simulink model "reactionWheel"  (R2019a)
settings: Solver=VariableStepAuto  StartTime=0.0  StopTime=20  RelTol=1e-3
model workspace (MAT data in the model file):
  Omega_max = 0.5
undefined symbols (not defined in the file or in its folder): sat, sigbuilder_block
libraries: simulink x3
settings Model: Creator=brice  LastModifiedBy=robin

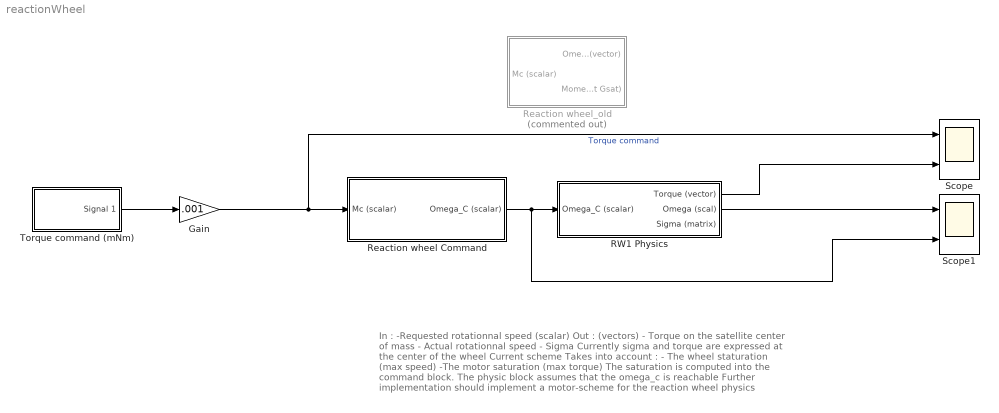
== system reactionWheel ==
  note: In :
      | -Requested rotationnal speed (scalar)
      | Out : (vectors)
      | - Torque on the satellite center of mass
      | - Actual rotationnal speed
      | - Sigma
      | Currently sigma and torque are expressed at the center of the wheel
      |
      | Current scheme
      | Takes into account :
      | - The wheel staturation (max speed)
      | -The motor saturation (max torque)
      |
      | The saturation is computed into the command block. The physic block assumes that the omega_c is reachable
      | Further implementation should implement a motor-scheme for the reaction wheel physics
  Gain : Gain  Gain=.001
  RW1 Physics : Subsystem
  Reaction wheel Command : Subsystem
  Reaction wheel_old : Subsystem  Commented=on
  Scope : Scope  NumInputPorts=2
  Scope1 : Scope  NumInputPorts=2
  Torque command (mNm) : Subsystem  Tag=STV Subsys  LoadFcn=sigbuilder_block('load');  StartFcn=sigbuilder_block('start');  StopFcn=sigbuilder_block('stop');  ClipboardFcn=sigbuilder_block('clipboard');  mask(Sigbuilder block){tuvar=[0:10]}
      mask help: Simulink:masks:SigbuilderBlock_MD
      mask init:
      | if ~strcmp(get_param(bdroot(gcbh),'SimulationStatus'),'stopped') tuvar = sigbuilder_block('maskInit'); end
      settings: CopyFcn=sigbuilder_block('copy');  DeleteFcn=sigbuilder_block('delete');  ModelCloseFcn=sigbuilder_block('modelClose');  PreSaveFcn=sigbuilder_block('preSave');  PauseFcn=sigbuilder_block('pause');  ContinueFcn=sigbuilder_block('continue');  NameChangeFcn=sigbuilder_block('namechange');  OpenFcn=sigbuilder_block('open',[437.6 199.2 604.15 400 ]);  CloseFcn=sigbuilder_block('close');
      mask Display: plot(0, 0, 100, 100,[2, 2, 32, 32, 2], [68, 8, 8, 68, 68],[32, 2], [38, 38], [32, 19, 2],[53, 60, 44], [32, 17, 17, 2],[16, 16, 31, 31]);txt = getActiveGroup(gcbh);text(2, 100, txt,'verticalAlignment', 'top');
  wires:
  Reaction wheel Command/1(Omega_C (scalar)) -> RW1 Physics/1(Omega_C (scalar)), Scope1/2
  Torque command (mNm)/1(Signal 1) -> Gain/1
  RW1 Physics/1(Torque (vector)) -> Scope/2
  Gain/1 -> Scope/1, Reaction wheel Command/1(Mc (scalar))  "Torque command"
  RW1 Physics/2(Omega (scal)) -> Scope1/1

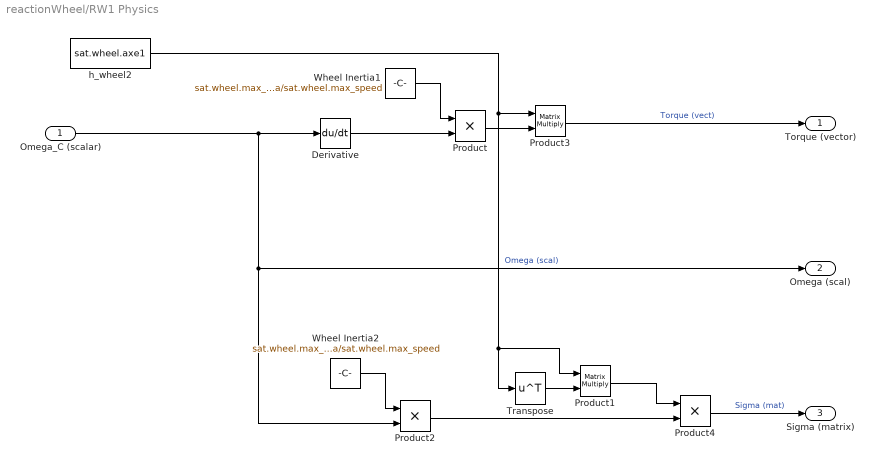
== system reactionWheel/RW1 Physics ==
  Omega_C (scalar) : Inport
  Derivative : Derivative
  Product : Product
  Product1 : Product  Multiplication=Matrix(*)
  Product2 : Product
  Product3 : Product  Multiplication=Matrix(*)
  Product4 : Product
  Transpose : Math  Operator=transpose  SaturateOnIntegerOverflow=on
  Wheel Inertia1 : Constant  Value=sat.wheel.max_sigma/sat.wheel.max_speed
  Wheel Inertia2 : Constant  Value=sat.wheel.max_sigma/sat.wheel.max_speed
  h_wheel2 : Constant  Value=sat.wheel.axe1
  Torque (vector) : Outport  VectorParamsAs1DForOutWhenUnconnected=on
  Omega (scal) : Outport  Port=2  VectorParamsAs1DForOutWhenUnconnected=on
  Sigma (matrix) : Outport  Port=3  VectorParamsAs1DForOutWhenUnconnected=on
  wires:
  Product3/1 -> Torque (vector)/1  "Torque (vect)"
  Wheel Inertia1/1 -> Product/1
  Omega_C (scalar)/1 -> Product2/2, Omega (scal)/1, Derivative/1  "Omega (scal)"
  Derivative/1 -> Product/2
  Product/1 -> Product3/2
  Wheel Inertia2/1 -> Product2/1
  Product4/1 -> Sigma (matrix)/1  "Sigma (mat)"
  Product2/1 -> Product4/2
  h_wheel2/1 -> Transpose/1, Product1/1, Product3/1
  Product1/1 -> Product4/1
  Transpose/1 -> Product1/2

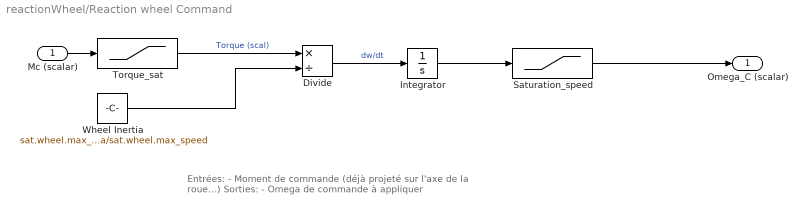
== system reactionWheel/Reaction wheel Command ==
  note: Entrées:
      | - Moment de commande (déjà projeté sur l'axe de la roue...)
      | Sorties:
      | - Omega de commande à appliquer
  Mc (scalar) : Inport
  Divide : Product  Inputs=*/
  Integrator : Integrator
  Saturation_speed : Saturate  UpperLimit=sat.wheel.max_speed  LowerLimit=- sat.wheel.max_speed
  Torque_sat : Saturate  UpperLimit=sat.wheel.max_torque  LowerLimit=- sat.wheel.max_torque
  Wheel Inertia : Constant  Value=sat.wheel.max_sigma/sat.wheel.max_speed
  Omega_C (scalar) : Outport  VectorParamsAs1DForOutWhenUnconnected=on
  wires:
  Mc (scalar)/1 -> Torque_sat/1
  Wheel Inertia/1 -> Divide/2
  Divide/1 -> Integrator/1  "dw/dt"
  Integrator/1 -> Saturation_speed/1
  Torque_sat/1 -> Divide/1  "Torque (scal)"
  Saturation_speed/1 -> Omega_C (scalar)/1

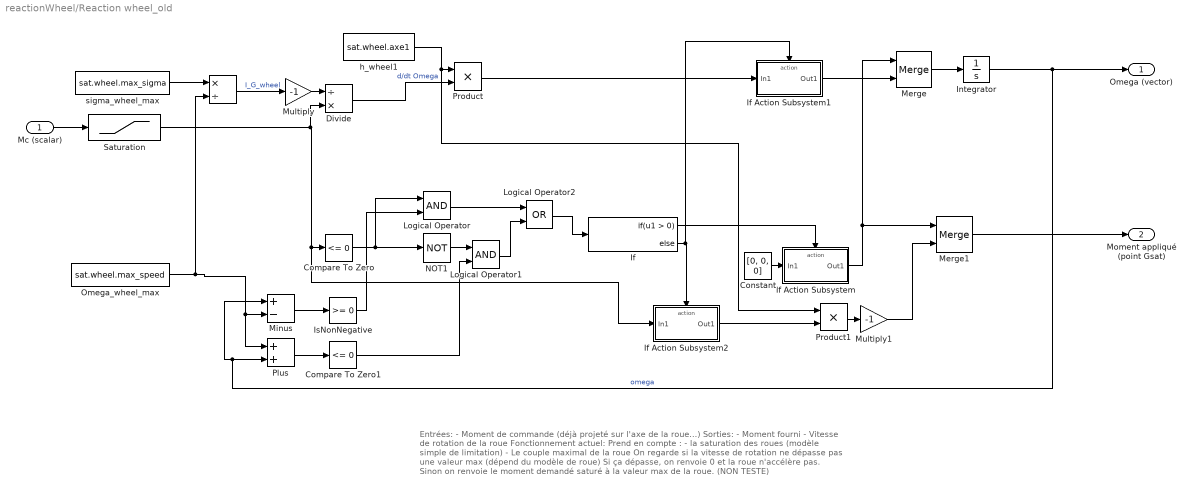
== system reactionWheel/Reaction wheel_old ==
  note: Entrées:
      | - Moment de commande (déjà projeté sur l'axe de la roue...)
      | Sorties:
      | - Moment fourni
      | - Vitesse de rotation de la roue
      |
      | Fonctionnement actuel:
      | Prend en compte :
      | - la saturation des roues (modèle simple de limitation)
      | - Le couple maximal de la roue
      |
      |
      | On regarde si la vitesse de rotation ne dépasse pas une valeur max (dépend du modèle de roue)
      | Si ça dépasse, on renvoie 0 et la roue n'accélère pas.
      | Sinon on renvoie le moment demandé saturé à la valeur max de la roue.
      |
      | (NON TESTE)
  Mc (scalar) : Inport
  " " : Product  Inputs=*/
  Compare To Zero : simulink/Logic and Bit Operations/Compare To Zero  relop=<=  OutDataTypeStr=boolean
  Compare To Zero1 : simulink/Logic and Bit Operations/Compare To Zero  relop=<=  OutDataTypeStr=boolean
  Constant : Constant  Value=[0, 0, 0]
  Divide : Product  Inputs=/*
  If : If
  If Action Subsystem : Subsystem  TreatAsAtomicUnit=on
  If Action Subsystem1 : Subsystem  TreatAsAtomicUnit=on
  If Action Subsystem2 : Subsystem  TreatAsAtomicUnit=on
  Integrator : Integrator
  IsNonNegative : simulink/Logic and Bit Operations/Compare To Zero  relop=>=  OutDataTypeStr=boolean
  Logical Operator : Logic  AllPortsSameDT=off  OutDataTypeStr=boolean
  Logical Operator1 : Logic  AllPortsSameDT=off  OutDataTypeStr=boolean
  Logical Operator2 : Logic  Operator=OR  AllPortsSameDT=off  OutDataTypeStr=boolean
  Merge : Merge
  Merge1 : Merge
  Minus : Sum  Inputs=+-
  Multiply : Gain  Gain=-1
  Multiply1 : Gain  Gain=-1
  NOT1 : Logic  Operator=NOT  IconShape=distinctive  AllPortsSameDT=off  OutDataTypeStr=boolean
  Omega_wheel_max : Constant  Value=sat.wheel.max_speed
  Plus : Sum
  Product : Product
  Product1 : Product
  Saturation : Saturate  UpperLimit=sat.wheel.max_torque  LowerLimit=- sat.wheel.max_torque
  h_wheel1 : Constant  Value=sat.wheel.axe1
  sigma_wheel_max : Constant  Value=sat.wheel.max_sigma
  Omega (vector) : Outport  VectorParamsAs1DForOutWhenUnconnected=on
  Moment appliqué (point Gsat) : Outport  Port=2  VectorParamsAs1DForOutWhenUnconnected=on
  wires:
  Integrator/1 -> Omega (vector)/1, Minus/1, Plus/2  "omega"
  If/2 -> If Action Subsystem2/Action, If Action Subsystem1/Action
  Saturation/1 -> If Action Subsystem2/1(In1), Compare To Zero/1, Divide/2
  IsNonNegative/1 -> Logical Operator/2
  Constant/1 -> If Action Subsystem/1(In1)
  Compare To Zero/1 -> Logical Operator/1, NOT1/1
  Divide/1 -> Product/2  "d/dt Omega"
  NOT1/1 -> Logical Operator1/1
  Omega_wheel_max/1 -> Plus/1, Minus/2, " "/2
  Logical Operator2/1 -> If/1
  If/1 -> If Action Subsystem/Action
  Product/1 -> If Action Subsystem1/1(In1)
  If Action Subsystem/1(Out1) -> Merge1/1, Merge/1
  Minus/1 -> IsNonNegative/1
  Compare To Zero1/1 -> Logical Operator1/2
  Plus/1 -> Compare To Zero1/1
  If Action Subsystem1/1(Out1) -> Merge/2
  Merge1/1 -> Moment appliqué (point Gsat)/1
  Logical Operator/1 -> Logical Operator2/1
  h_wheel1/1 -> Product1/1, Product/1
  Logical Operator1/1 -> Logical Operator2/2
  Multiply/1 -> Divide/1
  " "/1 -> Multiply/1  "I_G_wheel"
  sigma_wheel_max/1 -> " "/1
  Merge/1 -> Integrator/1
  Mc (scalar)/1 -> Saturation/1
  Product1/1 -> Multiply1/1
  Multiply1/1 -> Merge1/2
  If Action Subsystem2/1(Out1) -> Product1/2

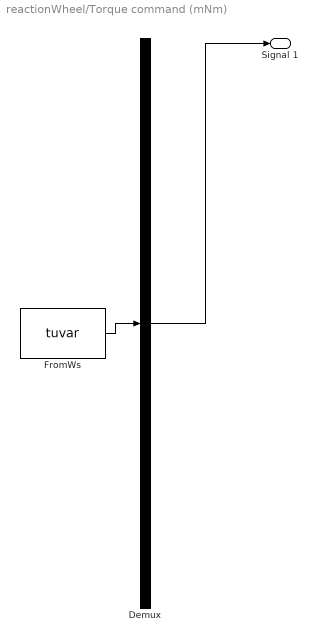
== system reactionWheel/Torque command (mNm) ==
  Demux : Demux  Tag=STV Demux  Outputs=1
  FromWs : FromWorkspace  Tag=STV FromWs  VariableName=tuvar  SampleTime=0
      SigBuilderData=|
      | common.afterFinalStr = 'Extrapolate'
      | common.sampleTime = 0
      | dataSet.timeRange = [0 20]
      | dataSet.name = 'Group 1'
      | sbobj.Groups.Name = 'Group 1'
      | sbobj.Groups.Signals.Name = 'Signal 1'
      | sbobj.Groups.Signals.XData = [0 4 4 6 6 7.95 7.95 10.05 10.05 10.7 10.7 19.2 19.2 20]
      | sbobj.Groups.Signals.YData = [0 0 1 1 0 0 1.395 1.395 0 0 1.89 1.89 0 0]
      | sbobj.Groups.TimeRange = [0 20]
  Signal 1 : Outport  Tag=STV Outport
  wires:
  Demux/1 -> Signal 1/1
  FromWs/1 -> Demux/1

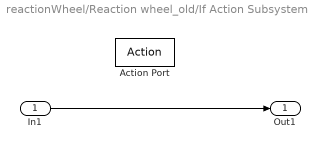
== system reactionWheel/Reaction wheel_old/If Action Subsystem ==
  In1 : Inport
  Action Port : ActionPort
  Out1 : Outport  VectorParamsAs1DForOutWhenUnconnected=on
  wires:
  In1/1 -> Out1/1

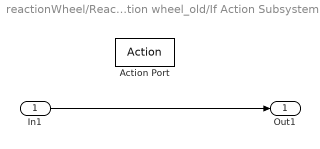
== system reactionWheel/Reaction wheel_old/If Action Subsystem1 ==
  In1 : Inport
  Action Port : ActionPort
  Out1 : Outport  VectorParamsAs1DForOutWhenUnconnected=on
  wires:
  In1/1 -> Out1/1

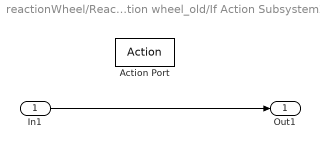
== system reactionWheel/Reaction wheel_old/If Action Subsystem2 ==
  In1 : Inport
  Action Port : ActionPort
  Out1 : Outport  VectorParamsAs1DForOutWhenUnconnected=on
  wires:
  In1/1 -> Out1/1
